simulink model "SlutgiltigaSystemet"  (R2018b)
settings: Solver=VariableStepAuto  StartTime=0.0  StopTime=10.0  RelTol=1e-3
values from neighbouring files (symbols this model uses):
  r_hjul = 0.05    [BB8parametrar.m]
  r_sfar = 0.25    [BB8parametrar.m]
libraries: simulink x1
settings Model: Creator=lampe  LastModifiedBy=lampe

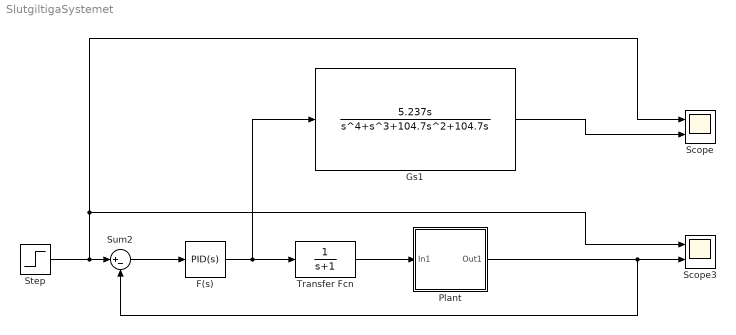
== system SlutgiltigaSystemet ==
  "F(s) " : simulink/Continuous/PID Controller  Controller=PID  Form=Parallel  TimeDomain=Continuous-time  SampleTime=-1  IntegratorMethod=Forward Euler  FilterMethod=Forward Euler  ControllerParametersSource=internal  P=3  I=18  D=0.6  UseFilter=on  N=75  TunerSelectOption=Transfer Function Based (PID Tuner App)  InitialConditionSource=internal  InitialConditionForIntegrator=0  InitialConditionForFilter=0  DifferentiatorICPrevScaledInput=0  ExternalReset=none  TrackingMode=off  Kt=1  LimitOutput=off  UpperSaturationLimit=inf  LowerSaturationLimit=-inf  LinearizeAsGain=on  AntiWindupMode=none  Kb=1  POutMin=[]  POutMax=[]  IOutMin=[]  IOutMax=[]  DOutMin=[]  DOutMax=[]  NOutMin=[]  NOutMax=[]  SumOutMin=[]  SumOutMax=[]  SaturationOutMin=[]  SaturationOutMax=[]  PParamMin=[]  PParamMax=[]  IParamMin=[]  IParamMax=[]  DParamMin=[]  DParamMax=[]  NParamMin=[]  NParamMax=[]  KbParamMin=[]  KbParamMax=[]  KtParamMin=[]  KtParamMax=[]  KbOutMin=[]  KbOutMax=[]  KtOutMin=[]  KtOutMax=[]  IntegratorOutMin=[]  IntegratorOutMax=[]  FilterOutMin=[]  FilterOutMax=[]  SumI1OutMin=[]  SumI1OutMax=[]  SumI2OutMin=[]  SumI2OutMax=[]  SumI3OutMin=[]  SumI3OutMax=[]  SumI4OutMin=[]  SumI4OutMax=[]  SumDOutMin=[]  SumDOutMax=[]  DifferentiatorOutMin=[]  DifferentiatorOutMax=[]  FilterDiffOutCoefMin=[]  FilterDiffOutCoefMax=[]  ReciprocalOutMin=[]  ReciprocalOutMax=[]  SumDenOutMin=[]  SumDenOutMax=[]  SumNumOutMin=[]  SumNumOutMax=[]  DivideOutMin=[]  DivideOutMax=[]  IntegratorContinuousStateAttributes=''  IntegratorStateMustResolveToSignalObject=off  IntegratorRTWStateStorageClass=Auto  FilterContinuousStateAttributes=''  FilterStateMustResolveToSignalObject=off  FilterRTWStateStorageClass=Auto  ParallelPVariant=InternalParameters  IdealPVariant=Disabled  IVariant=InternalParameters  DVariant=InternalParameters  IntegratorVariant=Continuous  SatVariant=Disabled  AWVariant=Passthrough  PCopyVariant=Disabled  TRVariant=Disabled  FdbkBlocksVariant=Forward  IdealPFdbkVariant=Disabled  SatFdbkVariant=Disabled  DerivativeFilterVariant=ContFilter  NVariant=InternalParameters  NCopyVariant=Disabled  FilterICVariant=InternalICsFilter  IntegratorICVariant=InternalICs  ExternalResetVariant=Disabled  TRSumVariant=Passthrough  SumFdbkVariant=Disabled  SumVariant=Sum_PID
  Gs1 : TransferFcn  Numerator=[5.237 0]  Denominator=[1 1 104.7 104.7 0]
  "Plant " : Subsystem
  Scope : Scope  NumInputPorts=2
  Scope3 : Scope  NumInputPorts=2
  Step : Step  SampleTime=0
  Sum2 : Sum  Inputs=|+-
  Transfer Fcn : TransferFcn  Denominator=[1 1]
  wires:
  Sum2/1 -> "F(s) "/1
  Step/1 -> Scope3/1, Scope/1, Sum2/1
  "Plant "/1(Out1) -> Sum2/2, Scope3/2
  Gs1/1 -> Scope/2
  "F(s) "/1 -> Transfer Fcn/1, Gs1/1
  Transfer Fcn/1 -> "Plant "/1(In1)

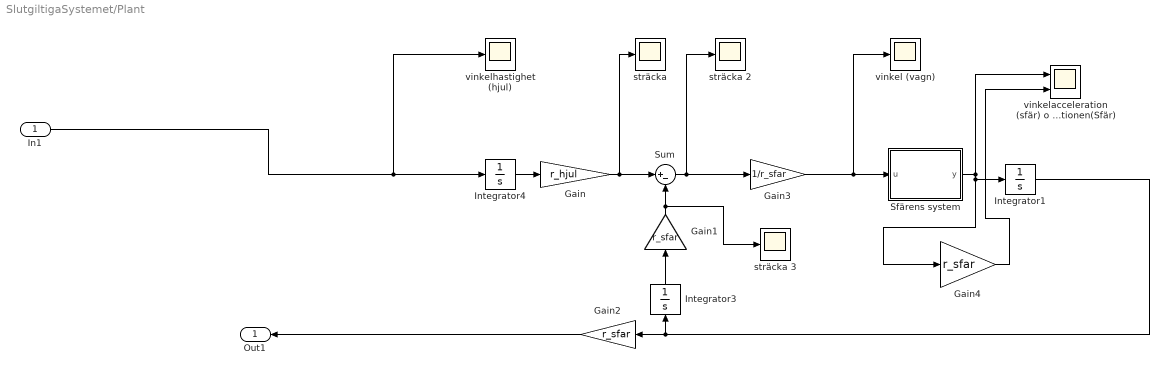
== system SlutgiltigaSystemet/Plant  ==
  In1 : Inport
  Gain : Gain  Gain=r_hjul
  Gain1 : Gain  Gain=r_sfar
  Gain2 : Gain  Gain=r_sfar
  Gain3 : Gain  Gain=1/r_sfar
  Gain4 : Gain  Gain=r_sfar
  Integrator1 : Integrator
  Integrator3 : Integrator
  Integrator4 : Integrator
  Sfärens system : MATLAB Function  TreatAsAtomicUnit=on
  Sum : Sum  Inputs=|+-
  sträcka : Scope
  "sträcka 2 " : Scope
  sträcka 3 : Scope
  vinkel (vagn) : Scope
  vinkelacceleration (sfär) o accelerationen(Sfär) : Scope  NumInputPorts=2
  vinkelhastighet (hjul) : Scope
  Out1 : Outport
  wires:
  Gain/1 -> Sum/1, sträcka/1
  Gain3/1 -> vinkel (vagn)/1, Sfärens system/1(u)
  Sum/1 -> Gain3/1, "sträcka 2 "/1
  Integrator1/1 -> Integrator3/1, Gain2/1
  Integrator4/1 -> Gain/1
  Gain1/1 -> sträcka 3/1, Sum/2
  Integrator3/1 -> Gain1/1
  Gain2/1 -> Out1/1
  In1/1 -> vinkelhastighet (hjul)/1, Integrator4/1
  Sfärens system/1(y) -> Gain4/1, Integrator1/1, vinkelacceleration (sfär) o accelerationen(Sfär)/1
  Gain4/1 -> vinkelacceleration (sfär) o accelerationen(Sfär)/2

== matlab function SlutgiltigaSystemet/Plant /Sfärens system ==
  data: u input; y output
function y = fcn(u)

r_sfar = 0.25; 
m_sfar = 3.3;  %byt till riktig
l_sfar = (2/3)*m_sfar*(r_sfar)^2 %Tröghetsshoffräs

m_innan = 8.0;%8.8 används i dagsläget %byt till riktig testa 2.0,8.0,16.0
F = m_innan*9.82;

mc = 2/3*r_sfar;       %centrums massa, position från centrum av sfären

phi = u %*pi/180

omega_prim = (sin(phi)*mc*F)/l_sfar

y = omega_prim;
